simulink library "Library_SII"  (R2014b)
settings: Solver=ode45  StartTime=0.0  StopTime=10.0  RelTol=1e-3
libraries: fl_lib x77, Library_SII x44, nesl_utility x33, powerlib x15, mblibv1 x11, simulink x6, elec_lib x5, powerlib_extras x1
(part 2 of 4)

== system Library_SII/Thermique ==
  Incidence surface : Subsystem  mask{lat=[45 46 46], lon=[-3 05 10], T_air=20, Hr=0.5, P_Atm=98232, B=0.1}
      mask prompts: lat "Latitude [°, ', '']"; lon "Longitude [°, ', '']"; T_air "Température de l'air (°C)"; Hr "Humidité relative"; P_Atm "Pression atmosphérique (Pa)"; B "Coefficient de trouble atmosphérique"
      mask help:
      | Coefficient de trouble atmosphérique
      | B = 0,02 pour un lieu situé en montagne
      | B = 0,05 pour un lieu rural
      | B = 0,10 pour un lieu urbain
      | B = 0,20 pour un lieu industriel (atmosphère polluée)
      mask Display:
      | [rgb, map, alpha] = imread('incidence.png', 'png');
      | image(rgb, [0.3, 0.05, 0.55, 0.7]);
      | port_label('input', 1, 'Energie soleil [W/m²]');
      | port_label('input', 3, 'Azimut soleil [°]');
      | port_label('input', 2, 'Hauteur soleil [°]');
      | port_label('input', 4, 'orientation surface [Nord = 0°]');
      | port_label('input', 5, 'inclinaison surface [Horiz = 0°]');
      | port_label('output', 1, 'Energie reçue [W/m²]');
  Paroi : Subsystem  mask(Paroi){m=Béton, d=off, lambda=0.92, c=880, mv=2200, s=1, e=10, Ti=20}
      mask prompts: m "Matériau"; d "Utiliser des valeurs personnalisées"; lambda "Conductivité thermique (W.m<sup>-1</sup>.K<sup>-1</sup>)"; c "Capacité thermique (J.kg<sup>-1</sup>.K<sup>-1</sup>)"; mv "Masse volumique (kg/m<sup>3</sup>)"; s "Surface de la paroi (m<sup>2</sup>)"; e "Epaisseur de la paroi (cm)"; Ti "Température initiale (°C)"
      mask help:
      | Modèle d'une paroi opaque (transmission de la chaleur par conduction).
      |
      | 1) Choisir un matériau
      | ou bien indiquer les caractéristiques thermiques d'un matériau
      | - Conductivité thermique (W.m-1.K-1)
      | - Capacité thermique (J.kg-1.K-1)
      | - Masse volumique (kg/m3)
      |
      | 2) Indiquer les dimensions de la paroi :
      | - Surface (m²)
      | - Epaisseur (cm)
      |
      | 3) Préciser la température initiale (°C)
      |
      | ==> Sortie :
      | T = Température au coeur de la paroi (°C)
      mask init:
      | % Conversion de la température
      | Ti = 273.15+Ti;
      | 
      | % Calcul de la masse
      | masse = mv * s * e / 100;
      | 
      | CaractMateriaux;
      mask Help:
      | Modèle d'une paroi opaque (transmission de la chaleur par conduction).
      | 
      | 1) Choisir un matériau
      | ou bien indiquer les caractéristiques thermiques d'un matériau
      | - Conductivité thermique (W.m<sup>-1</sup>.K<sup>-1</sup>)
      | - Capacité thermique (J.kg<sup>-1</sup>.K<sup>-1</sup>)
      | - Masse volumique (kg/m<sup>3</sup>)
      | 
      | 2) Indiquer les dimensions de la paroi :
      | - Surface (m²)
      | - Epaisseur (cm)
      | 
      | 3) Préciser la température initiale (°C)
      | 
      | ==> Sortie :
      | T = Température au coeur de la paroi (°C)
      | 
      | 
      | Il est possible de trouver les caractéristiques thermiques des principaux
      | matériaux de construction sur le site :
      | <a href="http://www.maison.com/architecture/maison-basse-consommation/quoi-construire-murs-maison-4881/"><tt>www.maison.com</tt></a>
      mask TypeOptions m: Shiste ardoise | Brique pleine | Béton | Béton armé | Béton cellulaire | Brique terre cuite pleine | Parpaing | Laine de verre | Laine de roche | Verre | Parpaing Monomur | PVC | Roche volcanique | Sapin | Panneau de particules agglomérées | Platre
      mask Callback m:
      | CaractMateriaux;
      | dd = get_param(gcb,'d');
      | if strcmp(dd,'off');
      |     mm =  get_param(gcb, 'm');
      |     set_param(gcb, 'lambda',Materiau(mm).Conductivite);
      |     set_param(gcb, 'mv',Materiau(mm).MasseVol);
      |     set_param(gcb, 'c',Materiau(mm).Capacite);
      | end
      mask Callback d:
      | maskStr = get_param(gcb,'MaskValues');
      | dd = get_param(gcb,'d');
      | if strcmp(dd,'on');
      |     set_param(gcb,'MaskEnables',{'on';'on';'on';'on';'on';'on';'on';'on'}),
      | else
      |     set_param(gcb,'MaskEnables',{'on';'on';'off';'off';'off';'on';'on';'on'}),
      | end
      mask Display:
      | image(imread(['Thermique/' Materiau(get_param(gcb, 'm')).Image]), [0.2, 0, 0.6, 0.85]);
      | port_label('lconn', 1, 'G');
      | port_label('rconn', 1, 'D');
      | port_label('output', 1, 'T');
      | 
      | 
      | text(0.5,0.95, get_param(gcb, 'm'), ...
      |      'HorizontalAlignment','center');
  Paroi (avec  rayonnement) : Subsystem  AncestorBlock=Library_SII/Thermique/Paroi (avec convection)  mask(Paroi){m=Parpaing, d=off, lambda=0.952, c=1080, mv=1185, s=200, e=10, Ti=20, Conv_Int=25, Conv_Ext=35}
      mask prompts: m "Matériau"; d "Utiliser des valeurs personnalisées"; lambda "Conductivité thermique (W.m<sup>-1</sup>.K<sup>-1</sup>)"; c "Capacité thermique (J.kg<sup>-1</sup>.K<sup>-1</sup>)"; mv "Masse volumique (kg/m<sup>3</sup>)"; s "Surface de la paroi (m<sup>2</sup>)"; e "Epaisseur de la paroi (cm)"; Ti "Température initiale (°C)"; Conv_Int "Coefficient de convection Intérieur (W/m²/K)"; Conv_Ext "Coefficient de convection Extérieur (W/m²/K)"
      mask help:
      | Modèle d'une paroi opaque. Transmission de la chaleur par :
      |  * conduction,
      |  * convection,
      |  * et rayonnement grace au port C.
      |
      | 1) Choisir un matériau
      | ou bien indiquer les caractéristiques thermiques d'un matériau
      | - Conductivité thermique [W.m-1.K-1]
      | - Capacité thermique [J.kg-1.K-1]
      | - Masse volumique [kg/m3]
      |
      | 2) Indiquer les dimensions de la paroi :
      | - Surface [m²]
      | - Epaisseur [cm]
      |
      | 3) Préciser la température initiale [°C]
      |
      | ==> Sortie :
      | T = Température au coeur de la paroi [°C]
      | F = Flux de chaleur traversant la paroi [W]
      mask init:
      | % Conversion de la température
      | Ti = 273.15+Ti;
      | 
      | % Calcul de la masse
      | masse = mv * s * e / 100;
      | 
      | CaractMateriaux;
      mask Help:
      | Modèle d'une paroi opaque (transmission de la chaleur par conduction).
      | 
      | 1) Choisir un matériau
      | ou bien indiquer les caractéristiques thermiques d'un matériau
      | - Conductivité thermique (W.m<sup>-1</sup>.K<sup>-1</sup>)
      | - Capacité thermique (J.kg<sup>-1</sup>.K<sup>-1</sup>)
      | - Masse volumique (kg/m<sup>3</sup>)
      | 
      | 2) Indiquer les dimensions de la paroi :
      | - Surface (m²)
      | - Epaisseur (cm)
      | 
      | 3) Préciser la température initiale (°C)
      | 
      | ==> Sortie :
      | T = Température au coeur de la paroi (°C)
      | 
      | 
      | Il est possible de trouver les caractéristiques thermiques des principaux
      | matériaux de construction sur le site :
      | <a href="http://www.maison.com/architecture/maison-basse-consommation/quoi-construire-murs-maison-4881/"><tt>www.maison.com</tt></a>
      mask TypeOptions m: Shiste ardoise | Brique pleine | Béton | Béton armé | Béton cellulaire | Brique terre cuite pleine | Parpaing | Laine de verre | Laine de roche | Verre | Parpaing Monomur | PVC | Roche volcanique | Sapin | Panneau de particules agglomérées | Platre
      mask Callback m:
      | CaractMateriaux;
      | dd = get_param(gcb,'d');
      | if strcmp(dd,'off');
      |     mm =  get_param(gcb, 'm');
      |     set_param(gcb, 'lambda',Materiau(mm).Conductivite);
      |     set_param(gcb, 'mv',Materiau(mm).MasseVol);
      |     set_param(gcb, 'c',Materiau(mm).Capacite);
      | end
      mask Callback d:
      | maskStr = get_param(gcb,'MaskValues');
      | dd = get_param(gcb,'d');
      | if strcmp(dd,'on');
      |     set_param(gcb,'MaskEnables',{'on';'on';'on';'on';'on';'on';'on';'on';'on';'on'}),
      | else
      |     set_param(gcb,'MaskEnables',{'on';'on';'off';'off';'off';'on';'on';'on';'on';'on'}),
      | end
      mask Display:
      | image(imread(['Thermique/' Materiau(get_param(gcb, 'm')).Image]), [0.2, 0, 0.6, 0.85]);
      | port_label('lconn', 1, 'Int');
      | port_label('rconn', 1, 'Ext');
      | port_label('rconn', 2, 'Ray');
      | port_label('output', 1, 'T');
      | port_label('output', 2, 'Fext');
      | port_label('output', 3, 'Fint');
      | 
      | 
      | text(0.5,0.95, get_param(gcb, 'm'), ...
      |      'HorizontalAlignment','center');
  Paroi (avec convection) : Subsystem  mask(Paroi){m=Parpaing, d=off, lambda=0.952, c=1080, mv=1185, s=200, e=10, Ti=20, Conv_Int=25, Conv_Ext=35}
      mask prompts: m "Matériau"; d "Utiliser des valeurs personnalisées"; lambda "Conductivité thermique (W.m<sup>-1</sup>.K<sup>-1</sup>)"; c "Capacité thermique (J.kg<sup>-1</sup>.K<sup>-1</sup>)"; mv "Masse volumique (kg/m<sup>3</sup>)"; s "Surface de la paroi (m<sup>2</sup>)"; e "Epaisseur de la paroi (cm)"; Ti "Température initiale (°C)"; Conv_Int "Coefficient de convection Intérieur (W/m²/K)"; Conv_Ext "Coefficient de convection Extérieur (W/m²/K)"
      mask help:
      | Modèle d'une paroi opaque (transmission de la chaleur par conduction).
      |
      | 1) Choisir un matériau
      | ou bien indiquer les caractéristiques thermiques d'un matériau
      | - Conductivité thermique (W.m-1.K-1)
      | - Capacité thermique (J.kg-1.K-1)
      | - Masse volumique (kg/m3)
      |
      | 2) Indiquer les dimensions de la paroi :
      | - Surface (m²)
      | - Epaisseur (cm)
      |
      | 3) Préciser la température initiale (°C)
      |
      | ==> Sortie :
      | T = Température au coeur de la paroi (°C)
      mask init:
      | % Conversion de la température
      | Ti = 273.15+Ti;
      | 
      | % Calcul de la masse
      | masse = mv * s * e / 100;
      | 
      | CaractMateriaux;
      mask Help:
      | Modèle d'une paroi opaque (transmission de la chaleur par conduction).
      | 
      | 1) Choisir un matériau
      | ou bien indiquer les caractéristiques thermiques d'un matériau
      | - Conductivité thermique (W.m<sup>-1</sup>.K<sup>-1</sup>)
      | - Capacité thermique (J.kg<sup>-1</sup>.K<sup>-1</sup>)
      | - Masse volumique (kg/m<sup>3</sup>)
      | 
      | 2) Indiquer les dimensions de la paroi :
      | - Surface (m²)
      | - Epaisseur (cm)
      | 
      | 3) Préciser la température initiale (°C)
      | 
      | ==> Sortie :
      | T = Température au coeur de la paroi (°C)
      | 
      | 
      | Il est possible de trouver les caractéristiques thermiques des principaux
      | matériaux de construction sur le site :
      | <a href="http://www.maison.com/architecture/maison-basse-consommation/quoi-construire-murs-maison-4881/"><tt>www.maison.com</tt></a>
      mask TypeOptions m: Shiste ardoise | Brique pleine | Béton | Béton armé | Béton cellulaire | Brique terre cuite pleine | Parpaing | Laine de verre | Laine de roche | Verre | Parpaing Monomur | PVC | Roche volcanique | Sapin | Panneau de particules agglomérées | Platre
      mask Callback m:
      | CaractMateriaux;
      | dd = get_param(gcb,'d');
      | if strcmp(dd,'off');
      |     mm =  get_param(gcb, 'm');
      |     set_param(gcb, 'lambda',Materiau(mm).Conductivite);
      |     set_param(gcb, 'mv',Materiau(mm).MasseVol);
      |     set_param(gcb, 'c',Materiau(mm).Capacite);
      | end
      mask Callback d:
      | maskStr = get_param(gcb,'MaskValues');
      | dd = get_param(gcb,'d');
      | if strcmp(dd,'on');
      |     set_param(gcb,'MaskEnables',{'on';'on';'on';'on';'on';'on';'on';'on';'on';'on'}),
      | else
      |     set_param(gcb,'MaskEnables',{'on';'on';'off';'off';'off';'on';'on';'on';'on';'on'}),
      | end
      mask Display:
      | image(imread(['Thermique/' Materiau(get_param(gcb, 'm')).Image]), [0.2, 0, 0.6, 0.85]);
      | port_label('lconn', 1, 'G');
      | port_label('rconn', 1, 'D');
      | port_label('output', 1, 'T');
      | 
      | 
      | text(0.5,0.95, get_param(gcb, 'm'), ...
      |      'HorizontalAlignment','center');
  Rayonnement solaire : Subsystem  mask{lat=[45 46 46], lon=[-3 05 10], T_air=20, Hr=0.5, P_Atm=98232, B=0.1}
      mask prompts: lat "Latitude [°, ', '']"; lon "Longitude [°, ', '']"; T_air "Température de l'air (°C)"; Hr "Humidité relative"; P_Atm "Pression atmosphérique (Pa)"; B "Coefficient de trouble atmosphérique"
      mask help:
      | Coefficient de trouble atmosphérique
      | B = 0,02 pour un lieu situé en montagne
      | B = 0,05 pour un lieu rural
      | B = 0,10 pour un lieu urbain
      | B = 0,20 pour un lieu industriel (atmosphère polluée)
      mask Display:
      | [rgb, map, alpha] = imread('Soleil.png', 'png');
      | image(rgb, [0.3, 0.1, 0.4, 0.8]);
      | port_label('input', 1, 'jour (1er janvier = 1)');
      | port_label('input', 2, 'heure [s] (minuit = 0s)');
      | port_label('output', 1, 'Energie soleil [W/m²]');
      | port_label('output', 3, 'Azimut soleil [°]');
      | port_label('output', 2, 'Hauteur soleil [°]');
  Vitrage : Subsystem  mask(Vitrage){typ=Simple, gaz=Air, itr=off, s=1, ev=4, evi=3.3, eg=6, egi=10, ev0=6, ege=10, eve=3.3, R=0.17181, U=5.8203, Ti=20}
      mask prompts: typ "Type de vitrage"; gaz "Type de gaz"; itr "Couche ITR"; s "Surface de la paroi (m<sup>2</sup>)"; ev "Epaisseur du verre (mm)"; evi "Epaisseur du verre intérieur (mm)"; eg "Epaisseur de la lame de gaz (mm)"; egi "Epaisseur de la lame de gaz coté intérieur (mm)"; ev0 "Epaisseur du verre intermédiaire (mm)"; ege "Epaisseur de la lame de gaz coté extérieur (mm)"; eve "Epaisseur du verre extérieur (mm)"; R "Résistance thermique (m².K/W)"; U "Coefficient thermique Ug (W/(m².K))"; Ti "Température initiale (°C)"
      mask help:
      | Modèle d'une vitre de fenêtre verticale.
      |
      | Type de vitrage : "Simple", "Double" ou "Triple"
      | Type de Gaz : le gaz remplissant les intervalles entre les parois de verre
      | Couche ITR = Isolation Thermique Renforcée : verre revêtu d'une couche
      | transparente d'oxydes métalliques nobles ou d'argent permettant
      | de retenir la chaleur à l'intérieur du logement.
      |
      | Ti et Te sont les températures de surfaces intérieure et extérieure.
      |
      | Résistance thermique et Coefficient Ug : ils caractérisent les transferts
      | thermiques à travers une paroi par conduction, convection et rayonnement.
      | L’ensemble de ces transferts thermiques est défini, selon la norme EN 673,
      | pour une vitesse de vent, des émissivités et des températures normalement
      | rencontrées dans le domaine du bâtiment.
      | (voir le document tarcog mathematical model.pdf pour plus de détails)
      mask init:
      | % Conversion de la température
      | %Ti = 273.15+Ti;
      | CaractMateriaux;
      | 
      | infini = '1e12';
      | sgaz = get_param(gcb, 'gaz');
      | sitr = get_param(gcb, 'itr');
      | switch typ
      |     case 1
      |         set_param([gcb '/Verre_int'], 'lambda', '1.2')
      |         set_param([gcb '/Verre_int'], 'e', num2str(ev))
      |         set_param([gcb '/Verre'], 'lambda', infini)
      |         set_param([gcb '/Verre_ext'], 'lambda', infini)
      |         set_param([gcb '/Gaz_int'], 'heat_tr_coeff', infini)
      |         set_param([gcb '/Gaz_ext'], 'heat_tr_coeff', infini)
      |    
      |     case 2
      |         set_param([gcb '/Verre_int'], 'lambda', '1.2')
      |         set_param([gcb '/Verre_int'], 'e', num2str(evi))
      |         set_param([gcb '/Verre'], 'lambda', infini)
      |         set_param([gcb '/Verre_ext'], 'lambda', '1.2')
      |         set_param([gcb '/Verre_ext'], 'e', num2str(eve))
      |         set_param([gcb '/Gaz_int'], 'heat_tr_coeff', calcul_conv_gaz(sgaz, num2str(eg), sitr, Materiau))
      |         set_param([gcb '/Gaz_ext'], 'heat_tr_coeff', infini)
      |         
      |     case 3
      |         set_param([gcb '/Verre_int'], 'lambda', '1.2')
      |         set_param([gcb '/Verre_int'], 'e', num2str(evi))
      |         set_param([gcb '/Verre'], 'lambda', '1.2')
      |         set_param([gcb '/Verre'], 'e', num2str(ev0))
      |         set_param([gcb '/Verre_ext'], 'lambda', '1.2')
      |         set_param([gcb '/Verre_ext'], 'e', num2str(eve))
      |         set_param([gcb '/Gaz_int'], 'heat_tr_coeff', calcul_conv_gaz(sgaz, num2str(egi), sitr, Materiau))
      |         set_param([gcb '/Gaz_ext'], 'heat_tr_coeff', calcul_conv_gaz(sgaz, num2str(ege), sitr, Materiau))
      | end
      mask TypeOptions typ: Simple | Double | Triple
      mask Callback typ:
      | CaractMateriaux;
      | typ = get_param(gcb, 'typ');
      | gaz = get_param(gcb, 'gaz');
      | itr = get_param(gcb, 'itr');
      | switch typ
      |     case 'Simple'
      |         set_param(gcb, 'MaskVisibilities',{'on';'off';'on';'on';'on';'off';'off';'off';'off';'off';'off';'on';'on';'on'})
      | 
      |     case 'Double'
      |         set_param(gcb, 'MaskVisibilities',{'on';'on';'on';'on';'off';'on';'on';'off';'off';'off';'on';'on';'on';'on'})
      | 
      |     case 'Triple'
      |         set_param(gcb, 'MaskVisibilities',{'on';'on';'on';'on';'off';'on';'off';'on';'on';'on';'on';'on';'on';'on'})
      | end
      | calcul_resistance(gcb, Materiau)
      mask TypeOptions gaz: Air | Argon
      mask Callback gaz: calcul_resistance(gcb, Materiau)
      mask Callback itr: calcul_resistance(gcb, Materiau)
      mask Callback ev:
      | if strcmp(typ, 'Simple')
      |     calcul_resistance(gcb, Materiau)
      | end
      mask Callback evi:
      | if not(strcmp(typ, 'Simple'))
      |     calcul_resistance(gcb, Materiau)
      | end
      mask Callback eg:
      | if strcmp(typ, 'Double')
      |     calcul_resistance(gcb, Materiau)
      | end
      mask Callback egi:
      | if strcmp(typ, 'Triple')
      |     calcul_resistance(gcb, Materiau)
      | end
      mask Callback ev0:
      | if strcmp(typ, 'Triple')
      |     calcul_resistance(gcb, Materiau)
      | end
      mask Callback ege:
      | if strcmp(typ, 'Triple')
      |     calcul_resistance(gcb, Materiau)
      | end
      mask Callback eve:
      | if not(strcmp(typ, 'Simple'))
      |     calcul_resistance(gcb, Materiau)
      | end
      mask Display:
      | CaractMateriaux;
      | image(imread(['Thermique/' Vitrage(get_param(gcb, 'typ')).Image]), [0.2, 0, 0.6, 0.85]);
      | port_label('lconn', 1, 'Int');
      | port_label('rconn', 1, 'Ext');
      | port_label('output', 1, 'T1');
      | port_label('output', 2, 'T2');
      | 
      | 
      | text(0.5,0.95, get_param(gcb, 'typ'), ...
      |      'HorizontalAlignment','center');

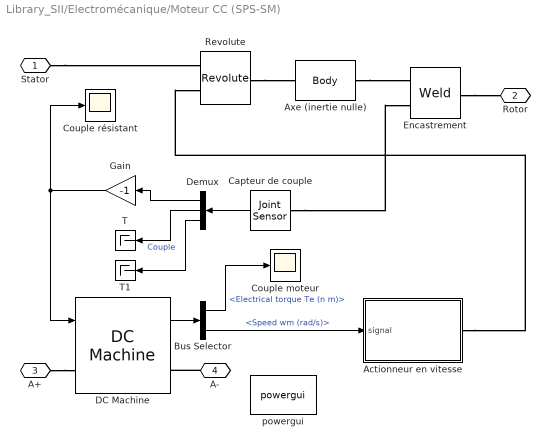
== system Library_SII/Electromécanique/Moteur CC (SPS-SM) ==
  Actionneur en vitesse : Subsystem
  Axe (inertie nulle) : mblibv1/Bodies/Body  LConnTagsString=CG  RConnTagsString=CS2  UpdateFromCAD=off  DialogClass=MechanicalBodyBlock  Mass=0.0001  MassUnits=kg  InertiaUnits=kg*m^2  Inertia=[1e-9 0 0 ; 0 1e-8 0 ; 0 0 1e-8]  Shape=Cylinder  ShapeDims=[1 1]  ShapeUnits=m  ShapeUse=false  Density=1  DensityUnits=kg/m^3  DensityUse=false  GraphicsMode=EQELLIPSE  BodyColorSelMode=COLORPALETTE  BodyColor=[0 1 0]  AttachedToCS=CG  CG=Left$CG$[0 0 0]$Adjoining$Adjoining$m$[0 0 0]$Euler X-Y-Z$deg$World$true$none  WorkingFrames=Right$CS2$[0 0 0]$CG$CG$mm$[0 0 0]$Euler X-Y-Z$deg$World$true$none  CGPos=[0 0 0]  CGRot=[0 0 0]  CS0Pos=[]  CS0Rot=[]  CS1Pos=[]  CS1Rot=[]  CS2Pos=[0 0 0]  CS2Rot=[0 0 0]  CS3Pos=[]  CS3Rot=[]  CS4Pos=[]  CS4Rot=[]  CS5Pos=[]  CS5Rot=[]  CS6Pos=[]  CS6Rot=[]  CS7Pos=[]  CS7Rot=[]  CS8Pos=[]  CS8Rot=[]  CS9Pos=[]  CS9Rot=[]  CS10Pos=[]  CS10Rot=[]  CS11Pos=[]  CS11Rot=[]  CS12Pos=[]  CS12Rot=[]  CS13Pos=[]  CS13Rot=[]  CS14Pos=[]  CS14Rot=[]  CS15Pos=[]  CS15Rot=[]  CS16Pos=[]  CS16Rot=[]  CS17Pos=[]  CS17Rot=[]  CS18Pos=[]  CS18Rot=[]  CS19Pos=[]  CS19Rot=[]  CS20Pos=[]  CS20Rot=[]
  Bus Selector : BusSelector  OutputSignals=Electrical torque Te (n m),Speed wm (rad/s)
  Capteur de couple : mblibv1/Sensors &  Actuators/Joint Sensor  UpdateFromCAD=off  PhysicalDomain=Mechanical  PortType=blob  Muxed=on  Pose=off  Angle=off  AngleUnits=deg  ArcVelocity=off  ArcVelocityUnits=deg/s  ArcAcceleration=off  ArcAccelerationUnits=deg/s^2  CoordPosition=on  CoordPositionUnits=m  Velocity=off  VelocityUnits=m/s  Acceleration=off  AccelerationUnits=m/s^2  Quaternion=on  QuaternionDT=off  QuaternionDDT=off  QuaternionUnits=off  OutputVector=[1]  ActiveIO=off  Width=3  DialogClass=MechanicalSensorBlock  Primitive=W  Force=off  ForceUnits=N  Torque=on  TorqueUnits=N*m  ReferenceFrame=Absolute (World)  ReactionSensedSide=Base  ReactionReferenceFrame=Absolute (World)  ReactionForce=off  ReactionForceUnits=N  ReactionMoment=on  ReactionMomentUnits=N*m
  Couple résistant : Scope
      settings: YMin=-0.0005  YMax=0.0065  MaxDataPoints=500000
  Couple moteur : Scope
      settings: SaveName=ScopeData3
  DC Machine : powerlib/Machines/DC Machine  PresetModel=No  MechanicalLoad=Torque TL  FieldType=Permanent magnet  ShowDetailedParameters=on  MeasurementBus=off  RLa=[R L]  RLf=[281.3 156]  Laf=0.9483  MachineConstant=Back-emf constant (V/rpm)  Ke=K  Kt=1.8  J=J  Bm=kv  Tf=kc  w0=0  Ifinit=1  TsPowergui=0  TsBlock=-1
      settings: AttributesFormatString=\n
  Demux : Demux  Outputs=3
  Encastrement : mblibv1/Joints/Weld  LConnTagsString=__newl0|SA1  RConnTagsString=__newr0  UpdateFromCAD=off  NumSAPorts=1  CutJoint=off  MarkAsCut=off  Primitives=weld  PrimitiveProps=W$World$[0 0 0]$weld  DialogClass=JointBlock  WAxis=[0 0 0]
  Gain : Gain  Gain=-1
  Revolute : mblibv1/Joints/Revolute  LConnTagsString=__newl0|SA1  RConnTagsString=__newr0  UpdateFromCAD=off  NumSAPorts=1  CutJoint=off  MarkAsCut=off  Primitives=prismatic  PrimitiveProps=R1$World$[1 0 0]$revolute  DialogClass=JointBlock  R1Axis=[1 0 0]
  T : Terminator
  T1 : Terminator
  powergui : powerlib/powergui  Priority=1  SimulationMode=Continuous  SolverType=Tustin  SampleTime=50e-3  frequency=60  SPID=off  DisableSnubberDevices=off  DisableRonSwitches=off  DisableVfSwitches=off  SwTol=0  DisplayEquations=off  Interpol=off  methode=off  Ts=100  frequencyindice=0  Pbase=100e6  ErrMax=1e-4  Iterations=50  UnitsV=kV  UnitsW=MW  FunctionMessages=off  echomessages=off  HookPort=off  EnableUseOfTLC=off  x0status=blocks  RestoreLinks=warning  ResistiveCurrentMeasurement=off  Frange=[0:2:500]  Ylog=off  Xlog=on  ShowGrid=off  save=off  variable=ZData  structure=0  ZoomFFT=off  StartTime=0.0  cycles=1  DisplayStyle=1  fundamental=60  FreqAxis=off  MaxFrequency=1000  frequencyindicesteady=1  RmsSteady=1  display=off
  Stator : PMIOPort  Port=1  Side=Left
  Rotor : PMIOPort  Port=2  Side=Right
  A+ : PMIOPort  Port=3  Side=Left
  A- : PMIOPort  Port=4  Side=Right
  wires:
  Bus Selector/2 -> Actionneur en vitesse/1(signal)  "<Speed wm (rad/s)>"
  Demux/3 -> T1/1
  Demux/2 -> T/1  "Couple"
  Demux/1 -> Gain/1
  Gain/1 -> Couple résistant/1, DC Machine/1
  Bus Selector/1 -> Couple moteur/1  "<Electrical torque Te (n m)>"
  Capteur de couple/1 -> Demux/1
  DC Machine/1 -> Bus Selector/1
  connections:
  A-/RConn1 -- DC Machine/RConn1
  A+/RConn1 -- DC Machine/LConn1
  Stator/RConn1 -- Revolute/LConn1
  Actionneur en vitesse/RConn1 -- Revolute/LConn2
  Encastrement/RConn1 -- Rotor/RConn1
  Capteur de couple/LConn1 -- Encastrement/LConn2
  Axe (inertie nulle)/RConn1 -- Encastrement/LConn1
  Revolute/RConn1 -- Axe (inertie nulle)/LConn1

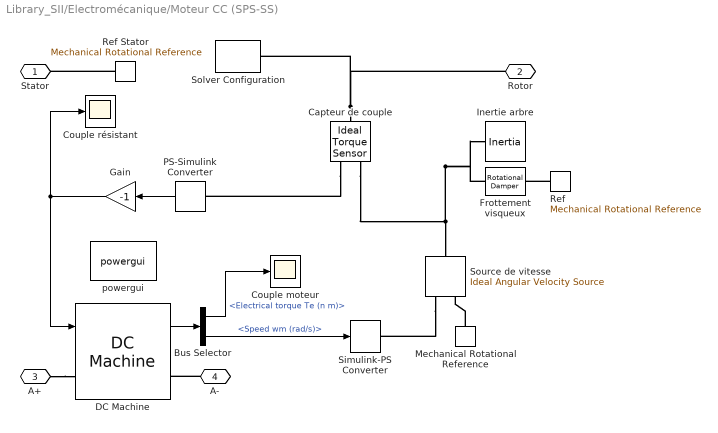
== system Library_SII/Electromécanique/Moteur CC (SPS-SS) ==
  Bus Selector : BusSelector  OutputSignals=Electrical torque Te (n m),Speed wm (rad/s)
  Capteur de couple : fl_lib/Mechanical/Mechanical Sensors/Ideal Torque Sensor
  Couple résistant : Scope
      settings: TimeRange=1  YMin=-0  YMax=0.0014  MaxDataPoints=500000
  Couple moteur : Scope
      settings: SaveName=ScopeData3
  DC Machine : powerlib/Machines/DC Machine  PresetModel=No  MechanicalLoad=Torque TL  FieldType=Permanent magnet  ShowDetailedParameters=on  MeasurementBus=off  RLa=[R L]  RLf=[281.3 156]  Laf=0.9483  MachineConstant=Back-emf constant (V/rpm)  Ke=K  Kt=1.8  J=J  Bm=kv  Tf=kc  w0=0  Ifinit=1  TsPowergui=0  TsBlock=-1
      settings: AttributesFormatString=\n
  Frottement visqueux : fl_lib/Mechanical/Rotational Elements/Rotational Damper  D=kv N*m/(rad/s)  w_specify=off  w_priority=High  w=0 rad/s  t_specify=off  t_priority=High  t=0 N*m
  Gain : Gain  Gain=-1
  Inertie arbre : fl_lib/Mechanical/Rotational Elements/Inertia  inertia=J kg*m^2  w_specify=on  w_priority=High  w=0 rad/s  t_specify=off  t_priority=High  t=0 N*m
  Mechanical Rotational Reference : fl_lib/Mechanical/Rotational Elements/Mechanical Rotational Reference
  PS-Simulink Converter : nesl_utility/PS-Simulink Converter  PhysicalDomain=network_engine_domain  SubClassName=ps_output  LeftPortType=input  RightPortType=output  PseudoPeriodic=off  Frequencies=[]  Unit=1  AffineConversion=off
  Ref : fl_lib/Mechanical/Rotational Elements/Mechanical Rotational Reference
  Ref Stator : fl_lib/Mechanical/Rotational Elements/Mechanical Rotational Reference
  Simulink-PS Converter : nesl_utility/Simulink-PS Converter  PhysicalDomain=network_engine_domain  SubClassName=ps_input  LeftPortType=input  RightPortType=output  PseudoPeriodic=off  Frequencies=[]  NoiseDistribution=none  NoiseParameters=[]  Unit=1  AffineConversion=off  InputFiltering=off  SimscapeFilterOrder=1  InputFilterTimeConstant=.001  UdotUserProvided=0
  Solver Configuration : nesl_utility/Solver Configuration  PhysicalDomain=network_engine_domain  SubClassName=solver  LeftPortType=input  RightPortType=generic  Accelerate=off  Tones=[]  Harmonics=[]  SimulateNoise=off  Profile=off  UseLocalSampling=off  EnableSwitchedLinearOptims=on  FrequencyDomain=off  UseCCode=off  RelTol=0.001  AbsTol=1e-06  MinStep=1e-09  ToWorkspace=off  DoDC=off  ResidualTolerance=1e-9  UseLocalSolver=off  LocalSolverChoice=NE_BACKWARD_EULER_ADVANCER  LocalSolverSampleTime=.001  DoFixedCost=off  MaxNonlinIter=3  MaxModeIter=2  LinearAlgebra=Sparse  DelaysMemoryBudget=1024  AutomaticFiltering=on  FilteringTimeConstant=0.001
  Source de vitesse : fl_lib/Mechanical/Mechanical Sources/Ideal Angular Velocity Source
  powergui : powerlib/powergui  Priority=1  SimulationMode=Continuous  SolverType=Tustin  SampleTime=50e-3  frequency=60  SPID=off  DisableSnubberDevices=off  DisableRonSwitches=off  DisableVfSwitches=off  SwTol=0  DisplayEquations=off  Interpol=off  methode=off  Ts=100  frequencyindice=0  Pbase=100e6  ErrMax=1e-4  Iterations=50  UnitsV=kV  UnitsW=MW  FunctionMessages=off  echomessages=off  HookPort=off  EnableUseOfTLC=off  x0status=blocks  RestoreLinks=warning  ResistiveCurrentMeasurement=off  Frange=[0:2:500]  Ylog=off  Xlog=on  ShowGrid=off  save=off  variable=ZData  structure=0  ZoomFFT=off  StartTime=0.0  cycles=1  DisplayStyle=1  fundamental=60  FreqAxis=off  MaxFrequency=1000  frequencyindicesteady=1  RmsSteady=1  display=off
  Stator : PMIOPort  Port=1  Side=Left
  Rotor : PMIOPort  Port=2  Side=Right
  A+ : PMIOPort  Port=3  Side=Left
  A- : PMIOPort  Port=4  Side=Right
  wires:
  Bus Selector/2 -> Simulink-PS Converter/1  "<Speed wm (rad/s)>"
  PS-Simulink Converter/1 -> Gain/1
  Gain/1 -> Couple résistant/1, DC Machine/1
  Bus Selector/1 -> Couple moteur/1  "<Electrical torque Te (n m)>"
  DC Machine/1 -> Bus Selector/1
  connections:
  Capteur de couple/RConn1 -- Source de vitesse/LConn1 -- Inertie arbre/LConn1 -- Frottement visqueux/RConn1
  Mechanical Rotational Reference/LConn1 -- Source de vitesse/RConn2
  Ref/LConn1 -- Frottement visqueux/LConn1
  Capteur de couple/LConn1 -- Solver Configuration/RConn1 -- Rotor/RConn1
  Capteur de couple/RConn2 -- PS-Simulink Converter/LConn1
  Ref Stator/LConn1 -- Stator/RConn1
  Source de vitesse/RConn1 -- Simulink-PS Converter/RConn1
  A-/RConn1 -- DC Machine/RConn1
  A+/RConn1 -- DC Machine/LConn1

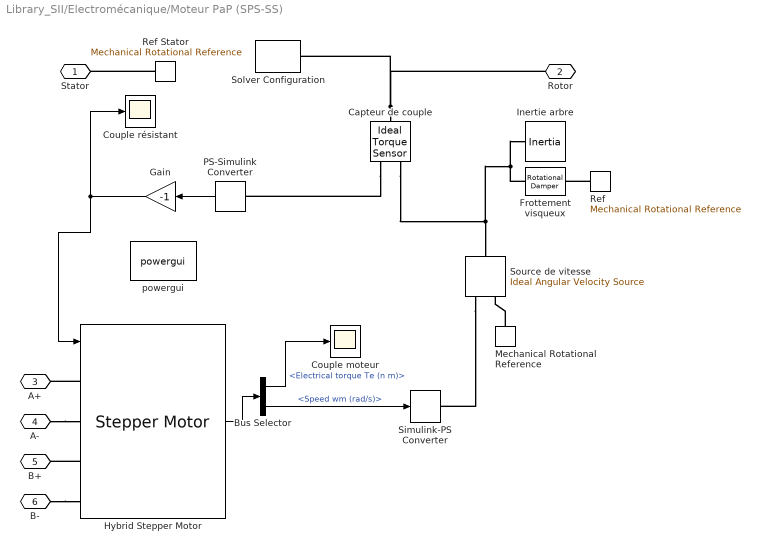
== system Library_SII/Electromécanique/Moteur PaP (SPS-SS) ==
  Bus Selector : BusSelector  OutputSignals=Electrical torque Te (n m),Speed wm (rad/s)
  Capteur de couple : fl_lib/Mechanical/Mechanical Sensors/Ideal Torque Sensor
  Couple résistant : Scope
      settings: TimeRange=1  YMin=-0  YMax=0.0014  MaxDataPoints=500000
  Couple moteur : Scope
      settings: SaveName=ScopeData3
  Frottement visqueux : fl_lib/Mechanical/Rotational Elements/Rotational Damper  D=kv N*m/(rad/s)  w_specify=off  w_priority=High  w=0 rad/s  t_specify=off  t_priority=High  t=0 N*m
  Gain : Gain  Gain=-1
  Hybrid Stepper Motor : powerlib/Machines/Stepper Motor  MotorType=Permanent-magnet / Hybrid  NumberOfPhases_1=2  NumberOfPhases_2=3  PresetModel_1=<empty>  PresetModel_2=<empty>  L=1.4e-3  Lmax=10e-3  Lmin=2e-3  R=0.7  Step_angle=1.8  Psim=0.005  Tdm=0.002  J=1.2e-7  B=1e-7*1000  w0=0  pos0=0  TsPowergui=0  TsBlock=-1
  Inertie arbre : fl_lib/Mechanical/Rotational Elements/Inertia  inertia=J kg*m^2  w_specify=on  w_priority=High  w=0 rad/s  t_specify=off  t_priority=High  t=0 N*m
  Mechanical Rotational Reference : fl_lib/Mechanical/Rotational Elements/Mechanical Rotational Reference
  PS-Simulink Converter : nesl_utility/PS-Simulink Converter  PhysicalDomain=network_engine_domain  SubClassName=ps_output  LeftPortType=input  RightPortType=output  PseudoPeriodic=off  Frequencies=[]  Unit=1  AffineConversion=off
  Ref : fl_lib/Mechanical/Rotational Elements/Mechanical Rotational Reference
  Ref Stator : fl_lib/Mechanical/Rotational Elements/Mechanical Rotational Reference
  Simulink-PS Converter : nesl_utility/Simulink-PS Converter  PhysicalDomain=network_engine_domain  SubClassName=ps_input  LeftPortType=input  RightPortType=output  PseudoPeriodic=off  Frequencies=[]  NoiseDistribution=none  NoiseParameters=[]  Unit=1  AffineConversion=off  InputFiltering=off  SimscapeFilterOrder=1  InputFilterTimeConstant=.001  UdotUserProvided=0
  Solver Configuration : nesl_utility/Solver Configuration  PhysicalDomain=network_engine_domain  SubClassName=solver  LeftPortType=input  RightPortType=generic  Accelerate=off  Tones=[]  Harmonics=[]  SimulateNoise=off  Profile=off  UseLocalSampling=off  EnableSwitchedLinearOptims=on  FrequencyDomain=off  UseCCode=off  RelTol=0.001  AbsTol=1e-06  MinStep=1e-09  ToWorkspace=off  DoDC=off  ResidualTolerance=1e-9  UseLocalSolver=off  LocalSolverChoice=NE_BACKWARD_EULER_ADVANCER  LocalSolverSampleTime=.001  DoFixedCost=off  MaxNonlinIter=3  MaxModeIter=2  LinearAlgebra=Sparse  DelaysMemoryBudget=1024  AutomaticFiltering=on  FilteringTimeConstant=0.001
  Source de vitesse : fl_lib/Mechanical/Mechanical Sources/Ideal Angular Velocity Source
  powergui : powerlib/powergui  Priority=1  SimulationMode=Continuous  SolverType=Tustin  SampleTime=50e-3  frequency=60  SPID=off  DisableSnubberDevices=off  DisableRonSwitches=off  DisableVfSwitches=off  SwTol=0  DisplayEquations=off  Interpol=off  methode=off  Ts=100  frequencyindice=0  Pbase=100e6  ErrMax=1e-4  Iterations=50  UnitsV=kV  UnitsW=MW  FunctionMessages=off  echomessages=off  HookPort=off  EnableUseOfTLC=off  x0status=blocks  RestoreLinks=warning  ResistiveCurrentMeasurement=off  Frange=[0:2:500]  Ylog=off  Xlog=on  ShowGrid=off  save=off  variable=ZData  structure=0  ZoomFFT=off  StartTime=0.0  cycles=1  DisplayStyle=1  fundamental=60  FreqAxis=off  MaxFrequency=1000  frequencyindicesteady=1  RmsSteady=1  display=off
  Stator : PMIOPort  Port=1  Side=Left
  Rotor : PMIOPort  Port=2  Side=Right
  A+ : PMIOPort  Port=3  Side=Left
  A- : PMIOPort  Port=4  Side=Right
  B+ : PMIOPort  Port=5  Side=Left
  B- : PMIOPort  Port=6  Side=Right
  wires:
  Bus Selector/2 -> Simulink-PS Converter/1  "<Speed wm (rad/s)>"
  PS-Simulink Converter/1 -> Gain/1
  Gain/1 -> Hybrid Stepper Motor/1, Couple résistant/1
  Bus Selector/1 -> Couple moteur/1  "<Electrical torque Te (n m)>"
  Hybrid Stepper Motor/1 -> Bus Selector/1
  connections:
  Capteur de couple/RConn1 -- Source de vitesse/LConn1 -- Frottement visqueux/RConn1 -- Inertie arbre/LConn1
  Mechanical Rotational Reference/LConn1 -- Source de vitesse/RConn2
  Ref/LConn1 -- Frottement visqueux/LConn1
  Capteur de couple/LConn1 -- Solver Configuration/RConn1 -- Rotor/RConn1
  Capteur de couple/RConn2 -- PS-Simulink Converter/LConn1
  Ref Stator/LConn1 -- Stator/RConn1
  Source de vitesse/RConn1 -- Simulink-PS Converter/RConn1
  A-/RConn1 -- Hybrid Stepper Motor/LConn2
  Hybrid Stepper Motor/LConn1 -- A+/RConn1
  Hybrid Stepper Motor/LConn3 -- B+/RConn1
  B-/RConn1 -- Hybrid Stepper Motor/LConn4

== system Library_SII/Electronique/Ampèremètre ==
  Current Sensor : fl_lib/Electrical/Electrical Sensors/Current Sensor
  S-PS : nesl_utility/PS-Simulink Converter  PhysicalDomain=network_engine_domain  SubClassName=ps_output  LeftPortType=input  RightPortType=output  PseudoPeriodic=off  Frequencies=[]  Unit=A  AffineConversion=off
  Conn1 : PMIOPort  Port=1  Side=Left
  Conn2 : PMIOPort  Port=2  Side=Right
  Out1 : Outport
  wires:
  S-PS/1 -> Out1/1
  connections:
  Current Sensor/RConn1 -- S-PS/LConn1
  Conn2/RConn1 -- Current Sensor/RConn2
  Conn1/RConn1 -- Current Sensor/LConn1

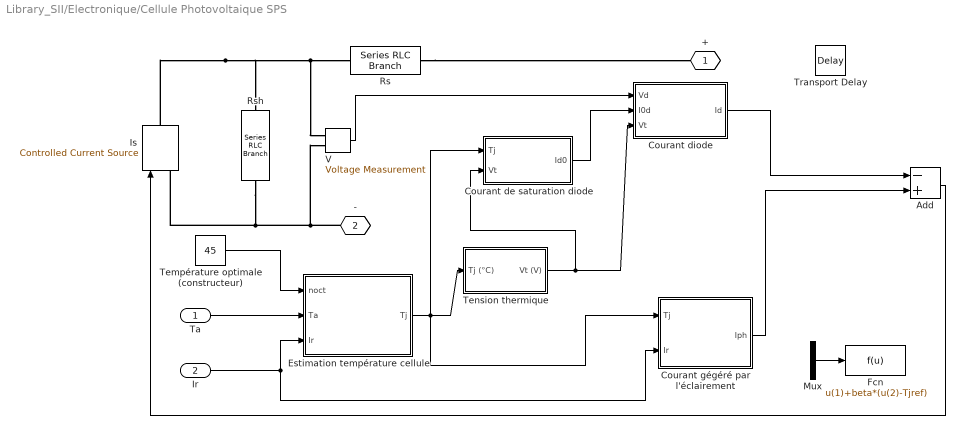
== system Library_SII/Electronique/Cellule Photovoltaique SPS ==
  Ta : Inport
  Ir : Inport  Port=2
  Add : Sum  Inputs=-+
  Courant de saturation diode : Subsystem
  Courant diode : Subsystem
  Courant gégéré par l'éclairement : Subsystem
  Estimation température cellule : Subsystem
  Fcn : Fcn  Expr=u(1)+beta*(u(2)-Tjref)
  Is : powerlib/Electrical Sources/Controlled Current Source  Initialize=on  Source_Type=AC  Amplitude=0  Phase=0  Frequency=0  Measurements=None
  Mux : Mux  Inputs=2
  Rs : powerlib/Elements/Series RLC Branch  LConnTagsString=__new0  RConnTagsString=__new0  BranchType=R  Resistance=Rs  Inductance=1e-3  SetiL0=off  InitialCurrent=0  Capacitance=1e-6  Setx0=off  InitialVoltage=0  Measurements=None
  Rsh : powerlib/Elements/Series RLC Branch  LConnTagsString=__new0  RConnTagsString=__new0  BranchType=R  Resistance=Rsh  Inductance=1e-3  SetiL0=off  InitialCurrent=0  Capacitance=1e-6  Setx0=off  InitialVoltage=0  Measurements=None
  Température optimale (constructeur) : Constant  Value=45
  Tension thermique : Subsystem
  Transport Delay : TransportDelay  DelayTime=0.001
  V : powerlib/Measurements/Voltage Measurement  PhasorSimulation=off  OutputType=Complex  PSBequivalent=0
  + : PMIOPort  Tag=PMCPort  Port=1  Side=Right
  - : PMIOPort  Tag=PMCPort  Port=2  Side=Right
  wires:
  Add/1 -> Is/1
  Estimation température cellule/1(Tj) -> Courant gégéré par l'éclairement/1(Tj), Tension thermique/1(Tj (°C)), Courant de saturation diode/1(Tj)
  Température optimale (constructeur)/1 -> Estimation température cellule/1(noct)
  Ta/1 -> Estimation température cellule/2(Ta)
  Ir/1 -> Estimation température cellule/3(Ir), Courant gégéré par l'éclairement/2(Ir)
  Courant gégéré par l'éclairement/1(Iph) -> Add/2
  Courant diode/1(Id) -> Add/1
  Mux/1 -> Fcn/1
  V/1 -> Courant diode/1(Vd)
  Tension thermique/1(Vt (V)) -> Courant diode/3(Vt), Courant de saturation diode/2(Vt)
  Courant de saturation diode/1(Id0) -> Courant diode/2(I0d)
  connections:
  V/LConn2 -- -/RConn1 -- Is/LConn1 -- Rsh/RConn1
  Is/RConn1 -- Rs/LConn1 -- V/LConn1 -- Rsh/LConn1
  Rs/RConn1 -- +/RConn1

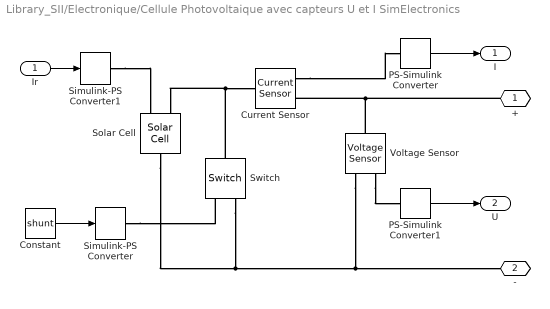
== system Library_SII/Electronique/Cellule Photovoltaique avec capteurs U et I SimElectronics ==
  Ir : Inport
  Constant : Constant  Value=shunt
  Current Sensor : fl_lib/Electrical/Electrical Sensors/Current Sensor
  PS-Simulink Converter : nesl_utility/PS-Simulink Converter  PhysicalDomain=network_engine_domain  SubClassName=ps_output  LeftPortType=input  RightPortType=output  PseudoPeriodic=off  Frequencies=[]  Unit=1  AffineConversion=off
  PS-Simulink Converter1 : nesl_utility/PS-Simulink Converter  PhysicalDomain=network_engine_domain  SubClassName=ps_output  LeftPortType=input  RightPortType=output  PseudoPeriodic=off  Frequencies=[]  Unit=1  AffineConversion=off
  Simulink-PS Converter : nesl_utility/Simulink-PS Converter  PhysicalDomain=network_engine_domain  SubClassName=ps_input  LeftPortType=input  RightPortType=output  PseudoPeriodic=off  Frequencies=[]  NoiseDistribution=none  NoiseParameters=[]  Unit=1  AffineConversion=off  InputFiltering=off  SimscapeFilterOrder=1  InputFilterTimeConstant=.001  UdotUserProvided=0
  Simulink-PS Converter1 : nesl_utility/Simulink-PS Converter  PhysicalDomain=network_engine_domain  SubClassName=ps_input  LeftPortType=input  RightPortType=output  PseudoPeriodic=off  Frequencies=[]  NoiseDistribution=none  NoiseParameters=[]  Unit=1  AffineConversion=off  InputFiltering=off  SimscapeFilterOrder=1  InputFilterTimeConstant=.001  UdotUserProvided=0
  Solar Cell : elec_lib/Sources/Solar Cell  prm=1  Isc=Icc A  Voc=Vco V  Is=1e-6 A  Is2=0 A  Iph=7.34 A  Ir0=IRef W/m^2  ec=Qf  N2=2  Rs=0 Ohm  Rp=Inf Ohm  N_series=1  TIPH1=0 1/K  EG=1.11 eV  TXIS1=3  TXIS2=3  TRS1=0  TRP1=0  Tmeas=TRef C  TFIXED=Tcell C  thermal_mass=100 J/K  initial_temperature=25 C
  Switch : fl_lib/Electrical/Electrical Elements/Switch  R_closed=1e-8 Ohm  G_open=1e-8 1/Ohm  Threshold=0  i_specify=off  i_priority=High  i=0 A  v_specify=off  v_priority=High  v=0 V
  Voltage Sensor : fl_lib/Electrical/Electrical Sensors/Voltage Sensor
  + : PMIOPort  Port=1  Side=Right
  - : PMIOPort  Port=2  Side=Right
  I : Outport
  U : Outport  Port=2
  wires:
  Ir/1 -> Simulink-PS Converter1/1
  PS-Simulink Converter/1 -> I/1
  PS-Simulink Converter1/1 -> U/1
  Constant/1 -> Simulink-PS Converter/1
  connections:
  Simulink-PS Converter1/RConn1 -- Solar Cell/LConn1
  Switch/RConn2 -- Voltage Sensor/RConn2 -- -/RConn1 -- Solar Cell/RConn1
  Voltage Sensor/LConn1 -- Current Sensor/RConn2 -- +/RConn1
  Voltage Sensor/RConn1 -- PS-Simulink Converter1/LConn1
  Current Sensor/RConn1 -- PS-Simulink Converter/LConn1
  Switch/LConn1 -- Current Sensor/LConn1 -- Solar Cell/LConn2
  Simulink-PS Converter/RConn1 -- Switch/RConn1

== system Library_SII/Electronique/Diode ==
  Tj (°C) : Inport
  Courant de saturation diode : Subsystem
  Courant diode : Subsystem
  Is : powerlib/Electrical Sources/Controlled Current Source  Initialize=on  Source_Type=AC  Amplitude=0  Phase=0  Frequency=0  Measurements=None
  Tension thermique : Subsystem
  V : powerlib/Measurements/Voltage Measurement  PhasorSimulation=off  OutputType=Complex  PSBequivalent=0
  C : PMIOPort  Tag=PMCPort  Port=1  Side=Right
  A : PMIOPort  Tag=PMCPort  Port=2  Side=Left
  wires:
  Courant diode/1(Id) -> Is/1
  V/1 -> Courant diode/1(Vd)
  Courant de saturation diode/1(Id0) -> Courant diode/2(I0d)
  Tj (°C)/1 -> Courant de saturation diode/1(Tj), Tension thermique/1(Tj (°C))
  Tension thermique/1(Vt) -> Courant diode/3(Vt)
  connections:
  Is/LConn1 -- C/RConn1 -- V/LConn2
  Is/RConn1 -- A/RConn1 -- V/LConn1

== system Library_SII/Electronique/Interrupteur ==
  In1 : Inport
  S-PS1 : nesl_utility/Simulink-PS Converter  PhysicalDomain=network_engine_domain  SubClassName=ps_input  LeftPortType=input  RightPortType=output  PseudoPeriodic=off  Frequencies=[]  NoiseDistribution=none  NoiseParameters=[]  Unit=1  AffineConversion=off  InputFiltering=off  SimscapeFilterOrder=1  InputFilterTimeConstant=.001  UdotUserProvided=0
  Switch : fl_lib/Electrical/Electrical Elements/Switch  R_closed=1e-8 Ohm  G_open=1e-8 1/Ohm  Threshold=0  i_specify=off  i_priority=High  i=0 A  v_specify=off  v_priority=High  v=0 V
  Conn1 : PMIOPort  Port=1  Side=Left
  Conn2 : PMIOPort  Port=2  Side=Right
  wires:
  In1/1 -> S-PS1/1
  connections:
  S-PS1/RConn1 -- Switch/RConn1
  Conn1/RConn1 -- Switch/LConn1
  Conn2/RConn1 -- Switch/RConn2
